simulink model "rotationmatrix"  (R2013a)
settings: Solver=ode3  StartTime=0.0  StopTime=2  FixedStep=1e-4  RelTol=1e-3
InitFcn:
  | k_d = 1.18e-7
  | B_a = 1.23e-6
  | u_min = 1.25
  | k_t = 3.7e-3
  | k_v = 7.8e-3
  | L_a = 1.9e-3
  | I_G = 1.5e-5
  | R_a = 260e-3
  | m = 0.694
  | l_a = 0.18
  | I_x = 5.87e-3
  | I_y = 5.87e-3
  | I_z = 10.73e-3
  | gamma0 = -47.7e-3
  | gamma1=1.3e-3
  | gamma2=-1.44e-6
  | gamma3=5.19e-4
  | g=9.8
  | delta_t=1e-4
libraries: cstblocks x8
settings Model: Creator=root  LastModifiedBy=root

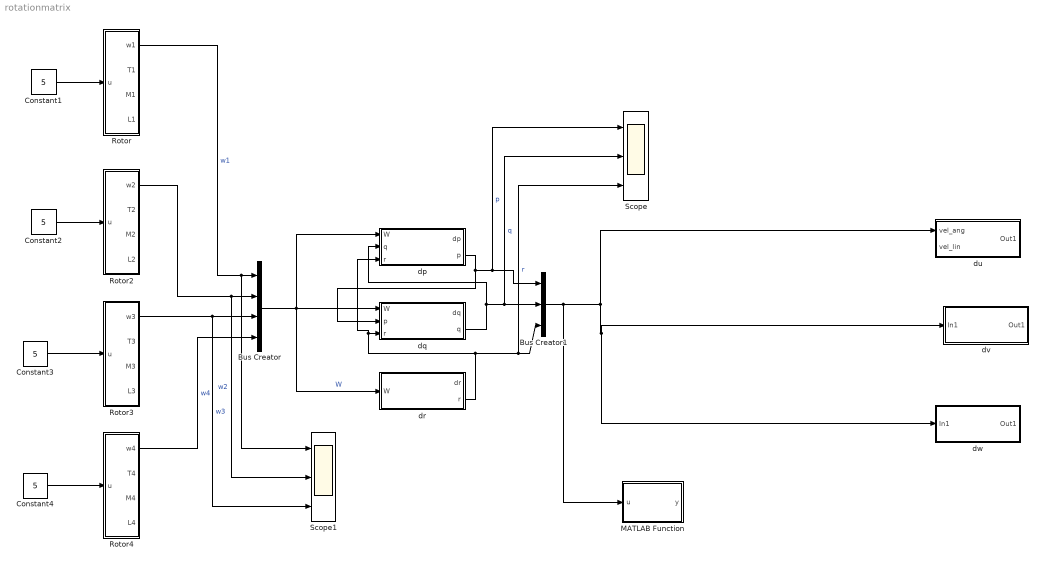
== system rotationmatrix ==
  Bus Creator : BusCreator
  Bus Creator1 : BusCreator  Inputs=3
  Constant{1..4} (4 alike) : Constant  Value=5
  MATLAB Function : MATLAB Function  TreatAsAtomicUnit=on
  Rotor : Subsystem
  Rotor2 : Subsystem
  Rotor3 : Subsystem
  Rotor4 : Subsystem
  Scope : Scope  NumInputPorts=3
      settings: YMin=-5~-5~-5  YMax=5~5~5
  Scope1 : Scope  NumInputPorts=3
      settings: YMin=-5~-5~-5  YMax=5~5~5  SaveName=ScopeData3
  dp : Subsystem
  dq : Subsystem
  dr : Subsystem
  du : Subsystem
  dv : Subsystem
  dw : Subsystem
  wires:
  Constant1/1 -> Rotor/1(u)
  Rotor2/1(w2) -> Scope1/2, Bus Creator/2  "w2"
  Rotor/1(w1) -> Scope1/1, Bus Creator/1  "w1"
  Rotor3/1(w3) -> Scope1/3, Bus Creator/3  "w3"
  Rotor4/1(w4) -> Bus Creator/4  "w4"
  Bus Creator/1 -> dp/1(W), dq/1(W), dr/1("W ")  "W"
  dp/2(p) -> Scope/1, Bus Creator1/1, dq/2("p ")  "p"
  dq/2(q) -> Scope/2, Bus Creator1/2, dp/2("q ")  "q"
  dr/2(r) -> Scope/3, Bus Creator1/3, dp/3(r), dq/3(r)  "r"
  Constant2/1 -> Rotor2/1(u)
  Constant3/1 -> Rotor3/1(u)
  Constant4/1 -> Rotor4/1(u)
  Bus Creator1/1 -> MATLAB Function/1(u), dw/1(In1), dv/1(In1), du/1(vel_ang)

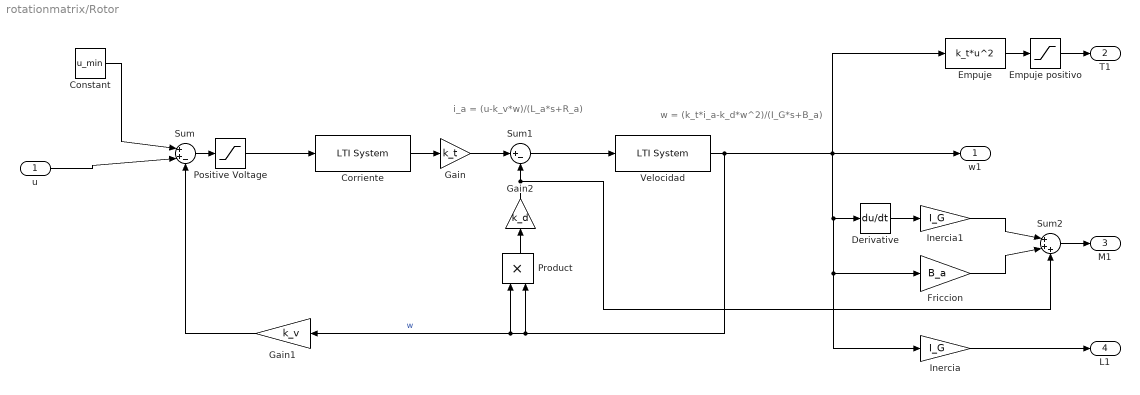
== system rotationmatrix/Rotor ==
  note: w = (k_t*i_a-k_d*w^2)/(I_G*s+B_a)
  note: i_a = (u-k_v*w)/(L_a*s+R_a)
  u : Inport
  Constant : Constant  Value=u_min
  Corriente : cstblocks/LTI System  sys=tf(1,[L_a R_a])  IC=[]
  Derivative : Derivative
  Empuje : Fcn  Expr=k_t*u^2
  Empuje positivo : Saturate  UpperLimit=inf  LowerLimit=0
  Friccion : Gain  Gain=B_a
  Gain : Gain  Gain=k_t
  Gain1 : Gain  Gain=k_v
  Gain2 : Gain  Gain=k_d
  Inercia : Gain  Gain=I_G
  Inercia1 : Gain  Gain=I_G
  Positive Voltage : Saturate  UpperLimit=30  LowerLimit=0
  Product : Product
  Sum : Sum  Inputs=|++-
  Sum1 : Sum  Inputs=|+-
  Sum2 : Sum  Inputs=|+++
  Velocidad : cstblocks/LTI System  sys=tf(1,[I_G B_a])  IC=[]
  w1 : Outport
  T1 : Outport  Port=2
  M1 : Outport  Port=3
  L1 : Outport  Port=4
  wires:
  Gain2/1 -> Sum2/3, Sum1/2
  Gain1/1 -> Sum/3
  Velocidad/1 -> Inercia/1, Friccion/1, Derivative/1, Empuje/1, w1/1, Product/2, Product/1, Gain1/1  "w"
  u/1 -> Sum/2
  Corriente/1 -> Gain/1
  Sum1/1 -> Velocidad/1
  Product/1 -> Gain2/1
  Sum/1 -> Positive Voltage/1
  Constant/1 -> Sum/1
  Positive Voltage/1 -> Corriente/1
  Gain/1 -> Sum1/1
  Empuje/1 -> Empuje positivo/1
  Empuje positivo/1 -> T1/1
  Derivative/1 -> Inercia1/1
  Inercia1/1 -> Sum2/1
  Friccion/1 -> Sum2/2
  Sum2/1 -> M1/1
  Inercia/1 -> L1/1

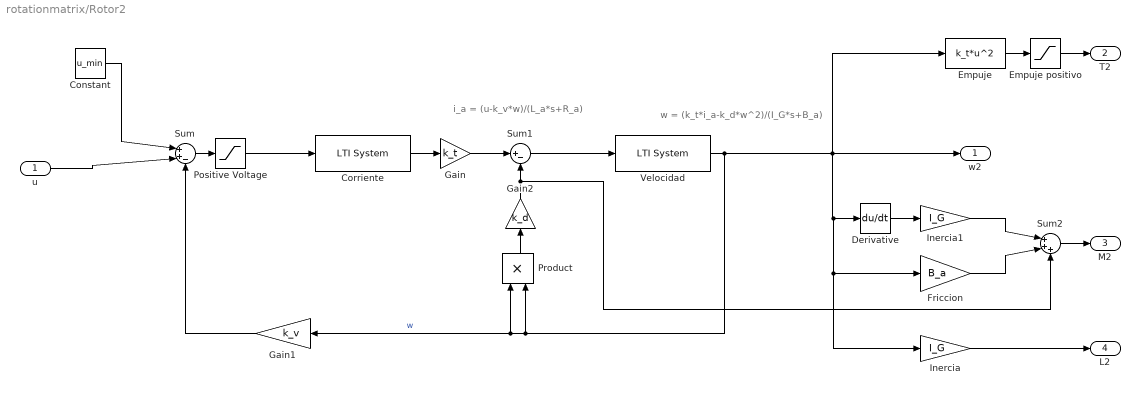
== system rotationmatrix/Rotor2 ==
  note: i_a = (u-k_v*w)/(L_a*s+R_a)
  note: w = (k_t*i_a-k_d*w^2)/(I_G*s+B_a)
  u : Inport
  Constant : Constant  Value=u_min
  Corriente : cstblocks/LTI System  sys=tf(1,[L_a R_a])  IC=[]
  Derivative : Derivative
  Empuje : Fcn  Expr=k_t*u^2
  Empuje positivo : Saturate  UpperLimit=inf  LowerLimit=0
  Friccion : Gain  Gain=B_a
  Gain : Gain  Gain=k_t
  Gain1 : Gain  Gain=k_v
  Gain2 : Gain  Gain=k_d
  Inercia : Gain  Gain=I_G
  Inercia1 : Gain  Gain=I_G
  Positive Voltage : Saturate  UpperLimit=30  LowerLimit=0
  Product : Product
  Sum : Sum  Inputs=|++-
  Sum1 : Sum  Inputs=|+-
  Sum2 : Sum  Inputs=|+++
  Velocidad : cstblocks/LTI System  sys=tf(1,[I_G B_a])  IC=[]
  w2 : Outport
  T2 : Outport  Port=2
  M2 : Outport  Port=3
  L2 : Outport  Port=4
  wires:
  Inercia/1 -> L2/1
  Sum2/1 -> M2/1
  Friccion/1 -> Sum2/2
  Inercia1/1 -> Sum2/1
  Derivative/1 -> Inercia1/1
  Empuje positivo/1 -> T2/1
  Empuje/1 -> Empuje positivo/1
  Gain/1 -> Sum1/1
  Positive Voltage/1 -> Corriente/1
  Constant/1 -> Sum/1
  Sum/1 -> Positive Voltage/1
  Product/1 -> Gain2/1
  Sum1/1 -> Velocidad/1
  Corriente/1 -> Gain/1
  u/1 -> Sum/2
  Velocidad/1 -> Gain1/1, Product/1, Product/2, w2/1, Empuje/1, Derivative/1, Friccion/1, Inercia/1  "w"
  Gain1/1 -> Sum/3
  Gain2/1 -> Sum1/2, Sum2/3

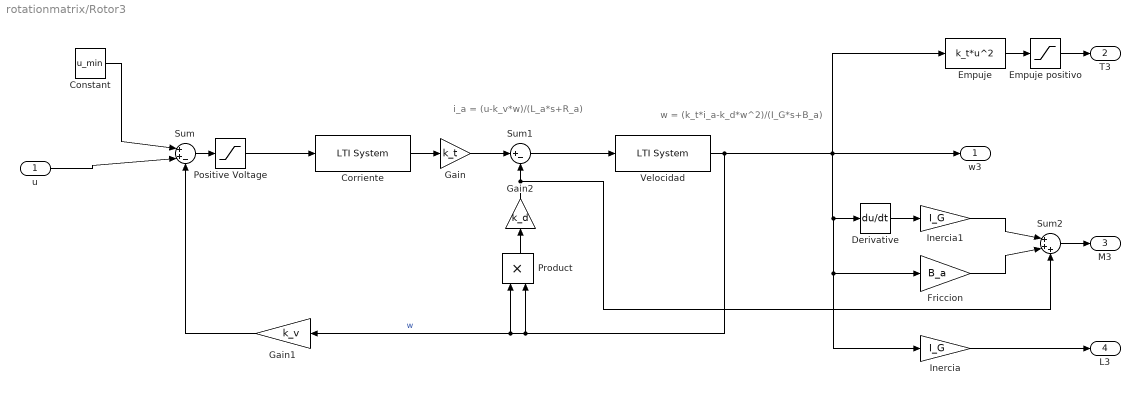
== system rotationmatrix/Rotor3 ==
  note: w = (k_t*i_a-k_d*w^2)/(I_G*s+B_a)
  note: i_a = (u-k_v*w)/(L_a*s+R_a)
  u : Inport
  Constant : Constant  Value=u_min
  Corriente : cstblocks/LTI System  sys=tf(1,[L_a R_a])  IC=[]
  Derivative : Derivative
  Empuje : Fcn  Expr=k_t*u^2
  Empuje positivo : Saturate  UpperLimit=inf  LowerLimit=0
  Friccion : Gain  Gain=B_a
  Gain : Gain  Gain=k_t
  Gain1 : Gain  Gain=k_v
  Gain2 : Gain  Gain=k_d
  Inercia : Gain  Gain=I_G
  Inercia1 : Gain  Gain=I_G
  Positive Voltage : Saturate  UpperLimit=30  LowerLimit=0
  Product : Product
  Sum : Sum  Inputs=|++-
  Sum1 : Sum  Inputs=|+-
  Sum2 : Sum  Inputs=|+++
  Velocidad : cstblocks/LTI System  sys=tf(1,[I_G B_a])  IC=[]
  w3 : Outport
  T3 : Outport  Port=2
  M3 : Outport  Port=3
  L3 : Outport  Port=4
  wires:
  Gain2/1 -> Sum2/3, Sum1/2
  Gain1/1 -> Sum/3
  Velocidad/1 -> Inercia/1, Friccion/1, Derivative/1, Empuje/1, w3/1, Product/2, Product/1, Gain1/1  "w"
  u/1 -> Sum/2
  Corriente/1 -> Gain/1
  Sum1/1 -> Velocidad/1
  Product/1 -> Gain2/1
  Sum/1 -> Positive Voltage/1
  Constant/1 -> Sum/1
  Positive Voltage/1 -> Corriente/1
  Gain/1 -> Sum1/1
  Empuje/1 -> Empuje positivo/1
  Empuje positivo/1 -> T3/1
  Derivative/1 -> Inercia1/1
  Inercia1/1 -> Sum2/1
  Friccion/1 -> Sum2/2
  Sum2/1 -> M3/1
  Inercia/1 -> L3/1

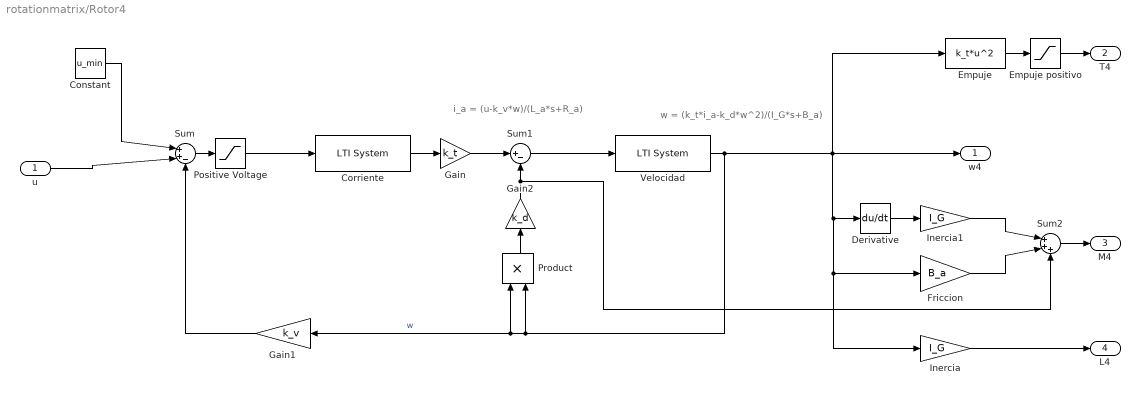
== system rotationmatrix/Rotor4 ==
  note: i_a = (u-k_v*w)/(L_a*s+R_a)
  note: w = (k_t*i_a-k_d*w^2)/(I_G*s+B_a)
  u : Inport
  Constant : Constant  Value=u_min
  Corriente : cstblocks/LTI System  sys=tf(1,[L_a R_a])  IC=[]
  Derivative : Derivative
  Empuje : Fcn  Expr=k_t*u^2
  Empuje positivo : Saturate  UpperLimit=inf  LowerLimit=0
  Friccion : Gain  Gain=B_a
  Gain : Gain  Gain=k_t
  Gain1 : Gain  Gain=k_v
  Gain2 : Gain  Gain=k_d
  Inercia : Gain  Gain=I_G
  Inercia1 : Gain  Gain=I_G
  Positive Voltage : Saturate  UpperLimit=30  LowerLimit=0
  Product : Product
  Sum : Sum  Inputs=|++-
  Sum1 : Sum  Inputs=|+-
  Sum2 : Sum  Inputs=|+++
  Velocidad : cstblocks/LTI System  sys=tf(1,[I_G B_a])  IC=[]
  w4 : Outport
  T4 : Outport  Port=2
  M4 : Outport  Port=3
  L4 : Outport  Port=4
  wires:
  Inercia/1 -> L4/1
  Sum2/1 -> M4/1
  Friccion/1 -> Sum2/2
  Inercia1/1 -> Sum2/1
  Derivative/1 -> Inercia1/1
  Empuje positivo/1 -> T4/1
  Empuje/1 -> Empuje positivo/1
  Gain/1 -> Sum1/1
  Positive Voltage/1 -> Corriente/1
  Constant/1 -> Sum/1
  Sum/1 -> Positive Voltage/1
  Product/1 -> Gain2/1
  Sum1/1 -> Velocidad/1
  Corriente/1 -> Gain/1
  u/1 -> Sum/2
  Velocidad/1 -> Gain1/1, Product/1, Product/2, w4/1, Empuje/1, Derivative/1, Friccion/1, Inercia/1  "w"
  Gain1/1 -> Sum/3
  Gain2/1 -> Sum1/2, Sum2/3

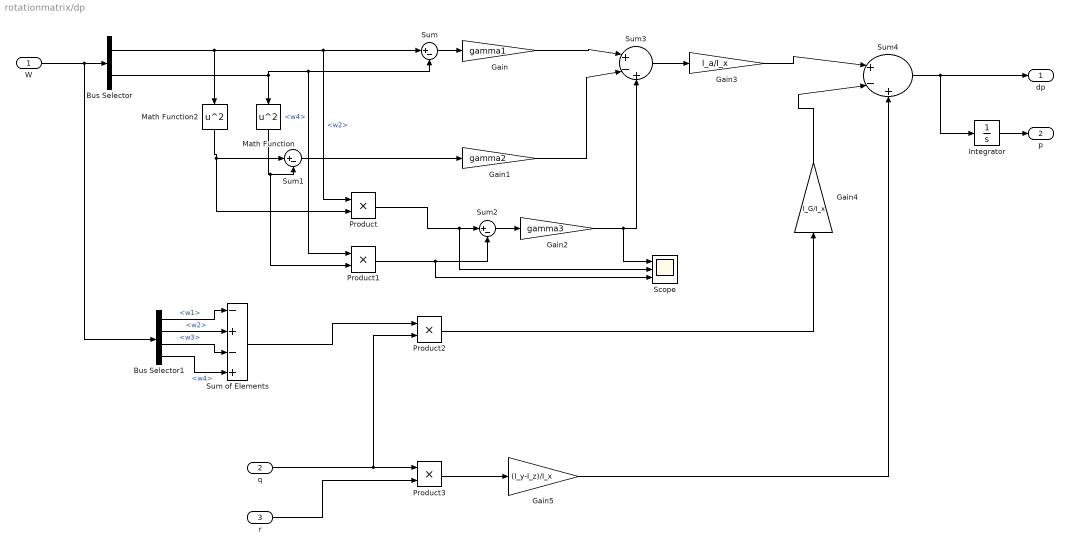
== system rotationmatrix/dp ==
  W : Inport
  "q " : Inport  Port=2
  r : Inport  Port=3
  Bus Selector : BusSelector  OutputSignals=w2,w4
  Bus Selector1 : BusSelector  OutputSignals=w1,w2,w3,w4
  Gain : Gain  Gain=gamma1
  Gain1 : Gain  Gain=gamma2
  Gain2 : Gain  Gain=gamma3
  Gain3 : Gain  Gain=l_a/I_x
  Gain4 : Gain  Gain=I_G/I_x
  Gain5 : Gain  Gain=(I_y-I_z)/I_x
  Integrator : Integrator
  Math Function : Math  Operator=square  SaturateOnIntegerOverflow=on
  Math Function2 : Math  Operator=square  SaturateOnIntegerOverflow=on
  Product{,1..3} (4 alike) : Product
  Scope : Scope  NumInputPorts=3
      settings: YMin=-5~-5~-5  YMax=5~5~5  SaveName=ScopeData2
  Sum : Sum  Inputs=|+-
  Sum of Elements : Sum  Inputs=-+-+
  Sum1 : Sum  Inputs=|+-
  Sum2 : Sum  Inputs=|+-
  Sum3 : Sum  Inputs=|+-+
  Sum4 : Sum  Inputs=|+-+
  dp : Outport
  p : Outport  Port=2
  wires:
  W/1 -> Bus Selector1/1, Bus Selector/1
  Bus Selector/1 -> Product/1, Sum/1, Math Function2/1  "<w2>"
  Bus Selector/2 -> Product1/1, Sum/2, Math Function/1  "<w4>"
  Sum/1 -> Gain/1
  Gain/1 -> Sum3/1
  Math Function2/1 -> Product/2, Sum1/1
  Math Function/1 -> Product1/2, Sum1/2
  Sum1/1 -> Gain1/1
  Product/1 -> Scope/2, Sum2/1
  Product1/1 -> Scope/3, Sum2/2
  Sum2/1 -> Gain2/1
  Gain1/1 -> Sum3/2
  Gain2/1 -> Scope/1, Sum3/3
  Sum3/1 -> Gain3/1
  Gain3/1 -> Sum4/1
  Gain4/1 -> Sum4/2
  Bus Selector1/1 -> Sum of Elements/1  "<w1>"
  Bus Selector1/2 -> Sum of Elements/2  "<w2>"
  Bus Selector1/3 -> Sum of Elements/3  "<w3>"
  Bus Selector1/4 -> Sum of Elements/4  "<w4>"
  Sum of Elements/1 -> Product2/1
  "q "/1 -> Product2/2, Product3/1
  Product2/1 -> Gain4/1
  r/1 -> Product3/2
  Product3/1 -> Gain5/1
  Gain5/1 -> Sum4/3
  Sum4/1 -> Integrator/1, dp/1
  Integrator/1 -> p/1

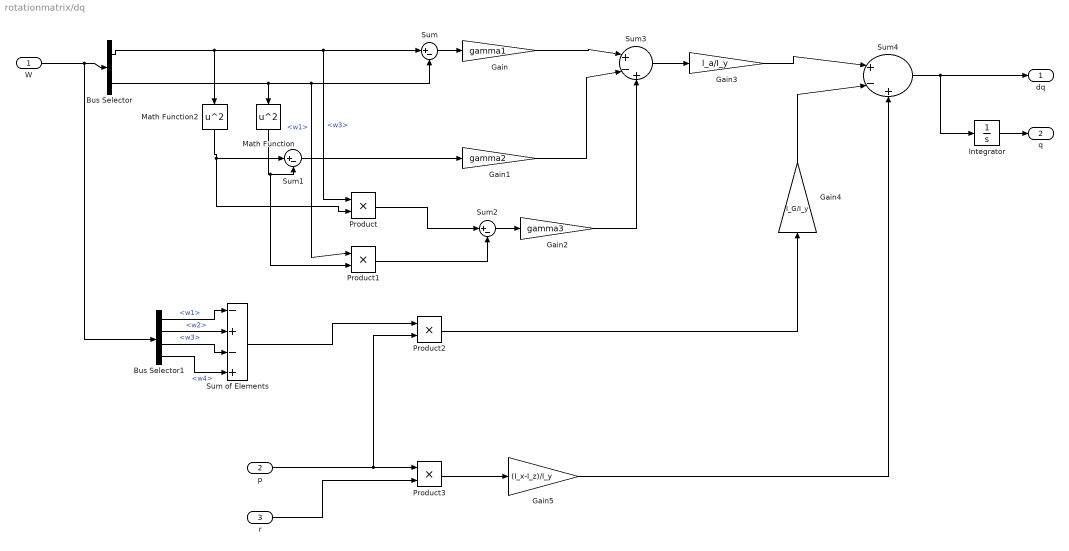
== system rotationmatrix/dq ==
  W : Inport
  "p " : Inport  Port=2
  r : Inport  Port=3
  Bus Selector : BusSelector  OutputSignals=w3,w1
  Bus Selector1 : BusSelector  OutputSignals=w1,w2,w3,w4
  Gain : Gain  Gain=gamma1
  Gain1 : Gain  Gain=gamma2
  Gain2 : Gain  Gain=gamma3
  Gain3 : Gain  Gain=l_a/I_y
  Gain4 : Gain  Gain=I_G/I_y
  Gain5 : Gain  Gain=(I_x-I_z)/I_y
  Integrator : Integrator
  Math Function : Math  Operator=square  SaturateOnIntegerOverflow=on
  Math Function2 : Math  Operator=square  SaturateOnIntegerOverflow=on
  Product{,1..3} (4 alike) : Product
  Sum : Sum  Inputs=|+-
  Sum of Elements : Sum  Inputs=-+-+
  Sum1 : Sum  Inputs=|+-
  Sum2 : Sum  Inputs=|+-
  Sum3 : Sum  Inputs=|+-+
  Sum4 : Sum  Inputs=|+-+
  dq : Outport
  q : Outport  Port=2
  wires:
  W/1 -> Bus Selector1/1, Bus Selector/1
  Bus Selector/1 -> Product/1, Sum/1, Math Function2/1  "<w3>"
  Sum/1 -> Gain/1
  Gain/1 -> Sum3/1
  Math Function2/1 -> Product/2, Sum1/1
  Sum1/1 -> Gain1/1
  Product/1 -> Sum2/1
  Sum2/1 -> Gain2/1
  Gain1/1 -> Sum3/2
  Gain2/1 -> Sum3/3
  Sum3/1 -> Gain3/1
  Gain4/1 -> Sum4/2
  Bus Selector1/1 -> Sum of Elements/1  "<w1>"
  Bus Selector1/2 -> Sum of Elements/2  "<w2>"
  Bus Selector1/3 -> Sum of Elements/3  "<w3>"
  Bus Selector1/4 -> Sum of Elements/4  "<w4>"
  Sum of Elements/1 -> Product2/1
  "p "/1 -> Product2/2, Product3/1
  Product2/1 -> Gain4/1
  r/1 -> Product3/2
  Product3/1 -> Gain5/1
  Gain5/1 -> Sum4/3
  Sum4/1 -> Integrator/1, dq/1
  Integrator/1 -> q/1
  Bus Selector/2 -> Product1/1, Sum/2, Math Function/1  "<w1>"
  Gain3/1 -> Sum4/1
  Math Function/1 -> Product1/2, Sum1/2
  Product1/1 -> Sum2/2

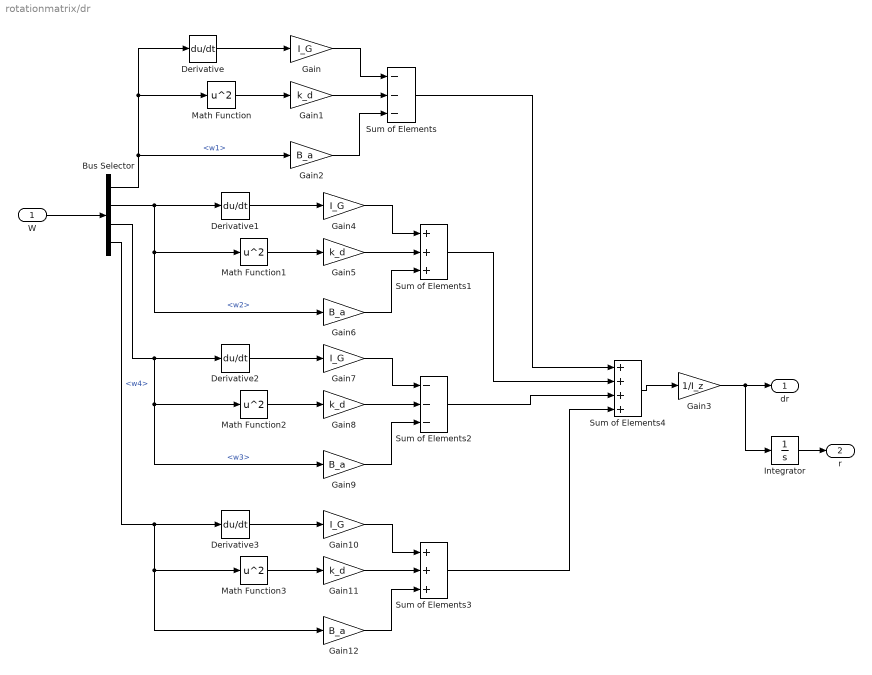
== system rotationmatrix/dr ==
  "W " : Inport
  Bus Selector : BusSelector  OutputSignals=w1,w2,w3,w4
  Derivative{,1..3} (4 alike) : Derivative
  Gain{,4,7,10} (4 alike) : Gain  Gain=I_G
  Gain{1,5,8,11} (4 alike) : Gain  Gain=k_d
  Gain{2,6,9,12} (4 alike) : Gain  Gain=B_a
  Gain3 : Gain  Gain=1/I_z
  Integrator : Integrator
  Math Function{,1..3} (4 alike) : Math  Operator=square  SaturateOnIntegerOverflow=on
  Sum of Elements : Sum  Inputs=---
  Sum of Elements1 : Sum  Inputs=+++
  Sum of Elements2 : Sum  Inputs=---
  Sum of Elements3 : Sum  Inputs=+++
  Sum of Elements4 : Sum  Inputs=++++
  dr : Outport
  r : Outport  Port=2
  wires:
  "W "/1 -> Bus Selector/1
  Derivative/1 -> Gain/1
  Bus Selector/1 -> Math Function/1, Derivative/1, Gain2/1  "<w1>"
  Math Function/1 -> Gain1/1
  Gain/1 -> Sum of Elements/1
  Gain1/1 -> Sum of Elements/2
  Gain2/1 -> Sum of Elements/3
  Sum of Elements/1 -> Sum of Elements4/1
  Derivative1/1 -> Gain4/1
  Bus Selector/2 -> Gain6/1, Math Function1/1, Derivative1/1  "<w2>"
  Math Function1/1 -> Gain5/1
  Gain4/1 -> Sum of Elements1/1
  Gain5/1 -> Sum of Elements1/2
  Gain6/1 -> Sum of Elements1/3
  Sum of Elements1/1 -> Sum of Elements4/2
  Derivative2/1 -> Gain7/1
  Bus Selector/3 -> Derivative2/1, Math Function2/1, Gain9/1  "<w3>"
  Math Function2/1 -> Gain8/1
  Gain7/1 -> Sum of Elements2/1
  Gain8/1 -> Sum of Elements2/2
  Gain9/1 -> Sum of Elements2/3
  Sum of Elements2/1 -> Sum of Elements4/3
  Derivative3/1 -> Gain10/1
  Bus Selector/4 -> Gain12/1, Math Function3/1, Derivative3/1  "<w4>"
  Math Function3/1 -> Gain11/1
  Gain10/1 -> Sum of Elements3/1
  Gain11/1 -> Sum of Elements3/2
  Gain12/1 -> Sum of Elements3/3
  Sum of Elements3/1 -> Sum of Elements4/4
  Sum of Elements4/1 -> Gain3/1
  Gain3/1 -> Integrator/1, dr/1
  Integrator/1 -> r/1

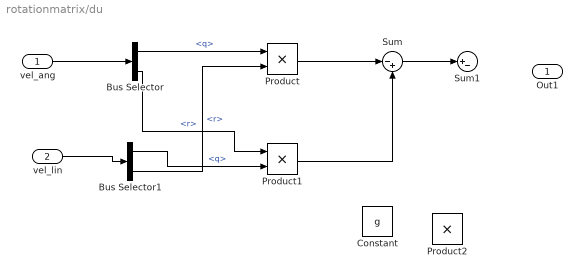
== system rotationmatrix/du ==
  vel_ang : Inport
  "vel_lin " : Inport  Port=2
  Bus Selector : BusSelector  OutputSignals=q,r
  Bus Selector1 : BusSelector  OutputSignals=q,r
  Constant : Constant  Value=g
  Product : Product
  Product1 : Product
  Product2 : Product
  Sum : Sum  Inputs=|-+
  Sum1 : Sum  Inputs=|+-
  Out1 : Outport
  wires:
  vel_ang/1 -> Bus Selector/1
  "vel_lin "/1 -> Bus Selector1/1
  Bus Selector/1 -> Product/1  "<q>"
  Bus Selector1/2 -> Product/2  "<r>"
  Bus Selector/2 -> Product1/1  "<r>"
  Bus Selector1/1 -> Product1/2  "<q>"
  Product/1 -> Sum/1
  Product1/1 -> Sum/2
  Sum/1 -> Sum1/1

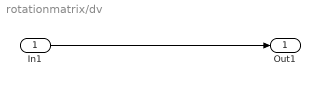
== system rotationmatrix/dv ==
  In1 : Inport
  Out1 : Outport
  wires:
  In1/1 -> Out1/1

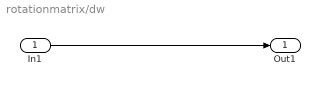
== system rotationmatrix/dw ==
  In1 : Inport
  Out1 : Outport
  wires:
  In1/1 -> Out1/1

== matlab function rotationmatrix/MATLAB Function ==
  data: u input; y output
function y = fcn(u)
%#codegen
%%
% Rotation matrix

w1 = u(1)
w2 = u(2)
w3 = u(3)
w4 = u(4)


y = u;
